simulink model "torqueBalancing2012b"  (Simulink 8.0)
settings: Solver=FixedStepDiscrete  StartTime=0.0  StopTime="CONFIG.SIMULATION_TIME "  FixedStep=CONFIG.Ts  RelTol=1e-3
InitFcn:
  | cd(fileparts(which(bdroot)));
  | initTorqueBalancing;
values from neighbouring files (symbols this model uses):
  WBT_modelName = 'matlabTorqueBalancing'    [initTorqueBalancing.m]
undefined symbols (not defined in the file or in its folder): bVectorConstraintsFeet, bVectorConstraintsLegs, CONFIG, ConstraintsMatrixFeet, ConstraintsMatrixLegs, DiscIntNeverNeededParam, gain, references, reg, ROBOT_DOF, ROBOT_DOF_FOR_SIMULINK, sat, SM, sm, WBT_robotName
libraries: WBToolboxLibrary x179, simulink x13
(part 1 of 4)
settings Model: Creator=daniele  LastModifiedBy=gnava
settings DebuggingCC: FcnCallInpInsideContextMsg=EnableAllAsWarning  FrameProcessingCompatibilityMsg=error
settings SFSimCC: SimParseCustomCode=off
settings CodeAppCC: CustomSymbolStrType=$N$R$M_T
settings GRTTargetCC: CodeReplacementLibrary=C89/C90 (ANSI)  CombineOutputUpdateFcns=off  GRTInterface=on

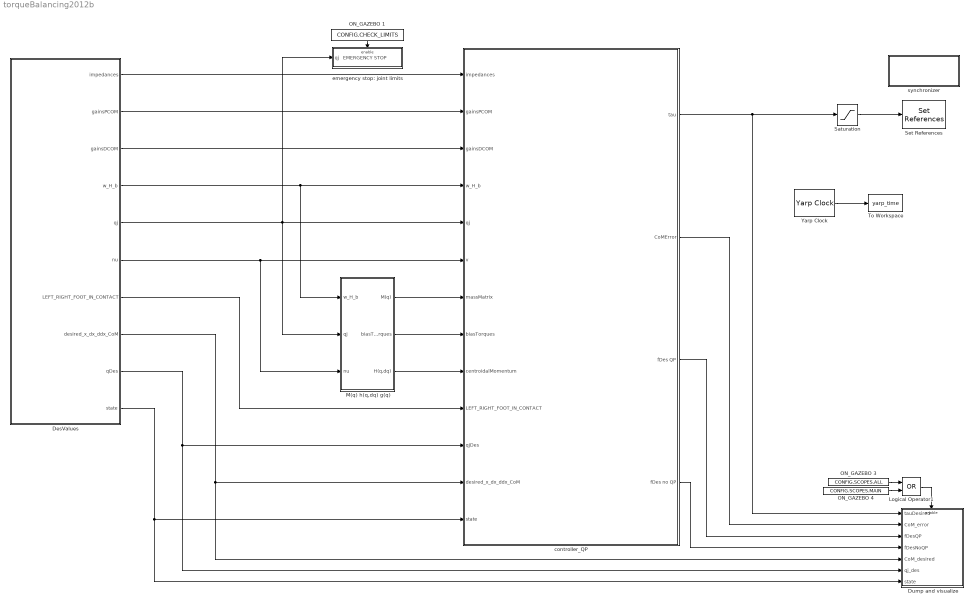
== system torqueBalancing2012b ==
  DesValues : Subsystem  Priority=-10
  Dump and visualize : Subsystem
  Logical Operator1 : Logic  Operator=OR  AllPortsSameDT=off  OutDataTypeStr=boolean
  M(q) h(q,dq) g(q) : Subsystem
  ON_GAZEBO 1 : Constant  Value=CONFIG.CHECK_LIMITS
  ON_GAZEBO 3 : Constant  Value=CONFIG.SCOPES.ALL
  ON_GAZEBO 4 : Constant  Value=CONFIG.SCOPES.MAIN
  Saturation : Saturate  UpperLimit=sat.torque  LowerLimit=-sat.torque
  Set References : WBToolboxLibrary/wholeBodyActuators/Set References  controlType=Torque  fullOrSubControl=Full  controlledJoints=''  robotName=WBT_robotName  localName=WBT_modelName  wbiFile=WBT_wbiFilename  wbiList=WBT_wbiList
  To Workspace : ToWorkspace  VariableName=yarp_time  SaveFormat=Structure With Time  SampleTime=-1
  Yarp Clock : WBToolboxLibrary/Utilities/Yarp Clock
  controller_QP : Subsystem
  emergency stop: joint limits : Subsystem
  synchronizer : Subsystem
      mask Display: disp('SYNCHRONIZER')
  wires:
  M(q) h(q,dq) g(q)/1(M(q)) -> controller_QP/7(massMatrix)
  DesValues/5(qj) -> emergency stop: joint limits/1(qj   EMERGENCY STOP), controller_QP/5(qj), M(q) h(q,dq) g(q)/2(qj)
  M(q) h(q,dq) g(q)/2(biasTorques) -> controller_QP/8(biasTorques)
  M(q) h(q,dq) g(q)/3(H(q,dq)) -> controller_QP/9(centroidalMomentum)
  controller_QP/1("tau ") -> Dump and visualize/1(tauDesired), Saturation/1
  controller_QP/2(CoMError) -> Dump and visualize/2(CoM_error)
  DesValues/9(qDes) -> Dump and visualize/6(qj_des), controller_QP/11(qjDes)
  DesValues/7(LEFT_RIGHT_FOOT_IN_CONTACT) -> controller_QP/10(LEFT_RIGHT_FOOT_IN_CONTACT)
  DesValues/8(desired_x_dx_ddx_CoM) -> controller_QP/12(desired_x_dx_ddx_CoM), Dump and visualize/5(CoM_desired)
  DesValues/1(impedances) -> controller_QP/1(impedances)
  Saturation/1 -> Set References/1
  DesValues/4(w_H_b) -> controller_QP/4(w_H_b), M(q) h(q,dq) g(q)/1(w_H_b)
  DesValues/6(nu) -> controller_QP/6(v), M(q) h(q,dq) g(q)/3(nu)
  Logical Operator1/1 -> Dump and visualize/Enable
  DesValues/10(state) -> Dump and visualize/7(state), controller_QP/13("state ")
  controller_QP/4(fDes no QP) -> Dump and visualize/4(fDesNoQP)
  controller_QP/3(fDes QP) -> Dump and visualize/3(fDesQP)
  ON_GAZEBO 1/1 -> emergency stop: joint limits/Enable
  ON_GAZEBO 3/1 -> Logical Operator1/1
  ON_GAZEBO 4/1 -> Logical Operator1/2
  DesValues/2(gainsPCOM) -> controller_QP/2(gainsPCOM)
  DesValues/3(gainsDCOM) -> controller_QP/3(gainsDCOM)
  Yarp Clock/1 -> To Workspace/1

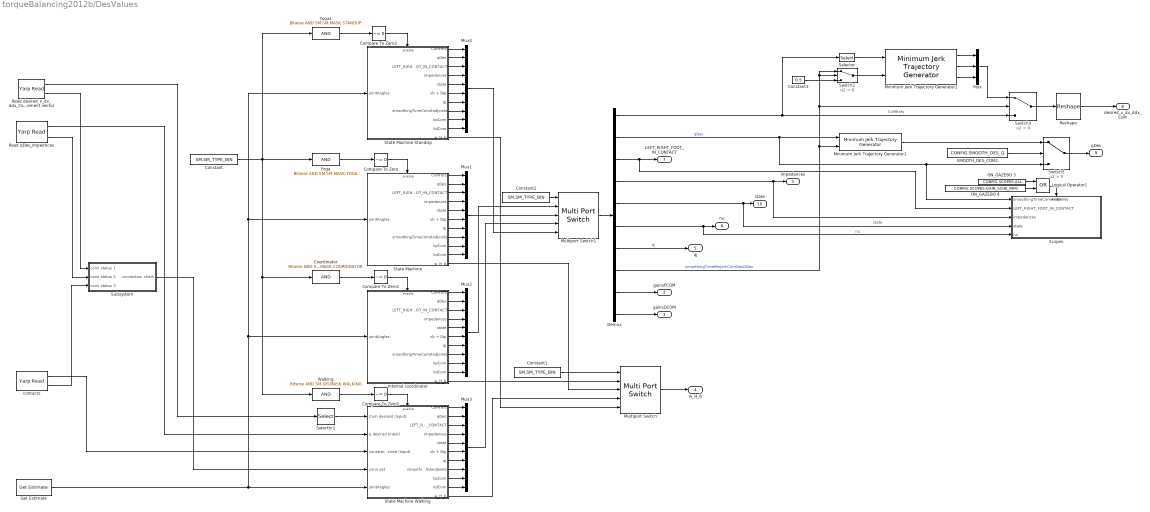
== system torqueBalancing2012b/DesValues ==
  Compare To Zero{,1..3} (4 alike) : simulink/Logic and Bit Operations/Compare To Zero  relop=~=  OutDataTypeStr=boolean
  Constant : Constant  Priority=-10  Value=SM.SM_TYPE_BIN  OutDataTypeStr=uint8
  Constant1 : Constant  Priority=-10  Value=SM.SM_TYPE_BIN  OutDataTypeStr=uint8
  Constant2 : Constant  Priority=-10  Value=SM.SM_TYPE_BIN  OutDataTypeStr=uint8
  Constant3 : Constant  Value=0.5
  Coordinator : simulink/Logic and Bit Operations/Bitwise Operator  logicop=AND  UseBitMask=on  BitMask=SM.SM.MASK.COORDINATOR  BitMaskRealWorld=Stored Integer
  Demux : Demux  Outputs=[9,ROBOT_DOF,2,ROBOT_DOF,1,ROBOT_DOF+6,ROBOT_DOF,1,3,3]
  Get Estimate : WBToolboxLibrary/wholeBodyStates/Get Estimate  estimateType=Joints Position  robotName=WBT_robotName  localName=WBT_modelName  wbiFile=WBT_wbiFilename  wbiList=WBT_wbiList
  Internal coordinator : Subsystem
  Logical Operator1 : Logic  Operator=OR  AllPortsSameDT=off  OutDataTypeStr=boolean
  Minimum Jerk Trajectory Generator1 : WBToolboxLibrary/Utilities/Minimum Jerk Trajectory Generator  externalSettlingTime=on  settlingTime=1  sampleTime=CONFIG.Ts  resetOnSettlingTime=off  firstDerivatives=off  secondDerivatives=off  explicitInitialValue=off
  Minimum Jerk Trajectory Generator2 : WBToolboxLibrary/Utilities/Minimum Jerk Trajectory Generator  externalSettlingTime=on  settlingTime=references.com.smoothingTime  sampleTime=CONFIG.Ts  resetOnSettlingTime=on  firstDerivatives=on  secondDerivatives=on  explicitInitialValue=off
  Multiport Switch : MultiPortSwitch  DataPortOrder=Specify indices  DataPortIndices={1, 2, 4, 6}
  Multiport Switch1 : MultiPortSwitch  DataPortOrder=Specify indices  DataPortIndices={1, 2, 4, 6}
  Mux : Mux  Inputs=3
  Mux{1..4} (4 alike) : Mux  Inputs=10
  ON_GAZEBO 3 : Constant  Value=CONFIG.SCOPES.ALL
  ON_GAZEBO 4 : Constant  Value=CONFIG.SCOPES.GAIN_SCHE_INFO
  Read desired_x_dx_ddx_CoM as 9 element vector : WBToolboxLibrary/Utilities/Yarp Read  portName=PORTS.COM_DES  signalSize=9  blocking=off  timestamp=off  autoconnect=off  errorOnConnection=on
  Read qDes_impednces : WBToolboxLibrary/Utilities/Yarp Read  portName=PORTS.Q_DES  signalSize=ROBOT_DOF  blocking=off  timestamp=off  autoconnect=off  errorOnConnection=on
  Reshape : Reshape  OutputDimensionality=Customize  OutputDimensions=[3,3]
  SMOOTH_DES_COM2 : Constant  Value=CONFIG.SMOOTH_DES_Q
  "Scopes  " : Subsystem
  Selector : Selector  InputPortWidth=9  IndexOptions=Index vector (dialog)  Indices=[1 2 3]  OutputSizes=1
  Selector1 : Selector  InputPortWidth=9  IndexOptions=Index vector (dialog)  Indices=[1 2 3]  OutputSizes=1
  State Machine : Subsystem  Priority=-100
  State Machine StandUp : Subsystem  Priority=-100
  State Machine Walking : Subsystem  Priority=-100
  Subsystem : Subsystem
  Switch1 : Switch  Criteria=u2 > Threshold
  Switch3 : Switch  Criteria=u2 > Threshold
  Switch5 : Switch  Criteria=u2 > Threshold
  Walking : simulink/Logic and Bit Operations/Bitwise Operator  logicop=AND  UseBitMask=on  BitMask=SM.SM.MASK.WALKING  BitMaskRealWorld=Stored Integer
  Yoga : simulink/Logic and Bit Operations/Bitwise Operator  logicop=AND  UseBitMask=on  BitMask=SM.SM.MASK.YOGA  BitMaskRealWorld=Stored Integer
  Yoga1 : simulink/Logic and Bit Operations/Bitwise Operator  logicop=AND  UseBitMask=on  BitMask=SM.SM.MASK.STANDUP  BitMaskRealWorld=Stored Integer
  contacts : WBToolboxLibrary/Utilities/Yarp Read  portName=['/' WBT_modelName '/constraints:i']  signalSize=2  blocking=off  timestamp=off  autoconnect=off  errorOnConnection=on
  impedances : Outport
  gainsPCOM : Outport  Port=2
  gainsDCOM : Outport  Port=3
  w_H_b : Outport  Port=4
  qj : Outport  Port=5
  nu : Outport  Port=6
  LEFT_RIGHT_FOOT_IN_CONTACT : Outport  Port=7
  desired_x_dx_ddx_CoM : Outport  Port=8
  qDes : Outport  Port=9
  state : Outport  Port=10
  wires:
  Read desired_x_dx_ddx_CoM as 9 element vector/2 -> Subsystem/1(conn status 1)
  Read desired_x_dx_ddx_CoM as 9 element vector/1 -> Selector1/1
  Reshape/1 -> desired_x_dx_ddx_CoM/1
  Read qDes_impednces/2 -> Subsystem/2(conn status 2)
  contacts/2 -> Subsystem/3(conn status 3)
  Switch3/1 -> Reshape/1
  SMOOTH_DES_COM2/1 -> Switch5/2
  Switch5/1 -> qDes/1
  Constant/1 -> Yoga1/1, Walking/1, Coordinator/1, Yoga/1
  State Machine/3(LEFT_RIGHT_FOOT_IN_CONTACT) -> Mux1/3
  State Machine/2(qDes) -> Mux1/2
  State Machine/1(CoMrefs) -> Mux1/1
  Internal coordinator/1(CoMrefs) -> Mux2/1
  Internal coordinator/2(qDes) -> Mux2/2
  Internal coordinator/3(LEFT_RIGHT_FOOT_IN_CONTACT) -> Mux2/3
  State Machine/4(impedances) -> Mux1/4
  Internal coordinator/4(impedances) -> Mux2/4
  State Machine/5(state) -> Mux1/5
  Internal coordinator/5(state) -> Mux2/5
  Internal coordinator/6(vb + Dqj) -> Mux2/6
  Internal coordinator/7(qj) -> Mux2/7
  State Machine/6(vb + Dqj) -> Mux1/6
  State Machine/7(qj) -> Mux1/7
  Demux/7 -> qj/1  "qj"
  State Machine Walking/4(impedances) -> Mux3/4
  State Machine Walking/3(LEFT_RIGHT_FOOT_IN_CONTACT) -> Mux3/3
  State Machine Walking/5(state) -> Mux3/5
  State Machine Walking/6(vb + Dqj) -> Mux3/6
  State Machine Walking/1(CoMrefs) -> Mux3/1
  State Machine Walking/7(qj) -> Mux3/7
  Coordinator/1 -> Compare To Zero1/1
  Yoga/1 -> Compare To Zero/1
  Walking/1 -> Compare To Zero2/1
  Mux3/1 -> Multiport Switch1/4
  Selector1/1 -> State Machine Walking/1(Com desired (input))
  Compare To Zero/1 -> State Machine/Enable
  Compare To Zero1/1 -> Internal coordinator/Enable
  Compare To Zero2/1 -> State Machine Walking/Enable
  Mux1/1 -> Multiport Switch1/3
  Mux2/1 -> Multiport Switch1/2
  State Machine/11(w_H_b) -> Multiport Switch/3
  Internal coordinator/11(w_H_b) -> Multiport Switch/2
  Read qDes_impednces/1 -> State Machine Walking/2(q desired (input))
  Subsystem/1(connection check) -> State Machine Walking/4(conn est)
  State Machine Walking/2(qDes) -> Mux3/2
  contacts/1 -> State Machine Walking/3(constraints desired (input))
  Multiport Switch/1 -> w_H_b/1
  Demux/5 -> state/1, "Scopes  "/4(state)  "state"
  Internal coordinator/8(smoothingTimeComAndJoints) -> Mux2/8
  State Machine Walking/8(smoothingTimeComAndJoints) -> Mux3/8
  State Machine/8(smoothingTimeComAndJoints) -> Mux1/8
  Demux/8 -> Switch1/1, Switch1/2, Switch3/2, Minimum Jerk Trajectory Generator1/2  "smoothingTimeMinJerkComDesQDes"
  Logical Operator1/1 -> "Scopes  "/Enable
  Demux/1 -> Selector/1, Switch3/3  "CoMRefs"
  Demux/2 -> Minimum Jerk Trajectory Generator1/1, "Scopes  "/1(smoothingTimeComAndJoints), Switch5/3  "qDes"
  Minimum Jerk Trajectory Generator1/1 -> Switch5/1
  ON_GAZEBO 3/1 -> Logical Operator1/1
  ON_GAZEBO 4/1 -> Logical Operator1/2
  Demux/6 -> nu/1, "Scopes  "/5(nu)  "nu"
  State Machine/9(kpCom) -> Mux1/9
  State Machine/10(kdCom) -> Mux1/10
  Internal coordinator/9(kpCom) -> Mux2/9
  Internal coordinator/10(kdCom) -> Mux2/10
  State Machine Walking/9(kpCom) -> Mux3/9
  State Machine Walking/10(kdCom) -> Mux3/10
  Multiport Switch1/1 -> Demux/1
  Demux/4 -> impedances/1, "Scopes  "/3(impedances)
  Demux/3 -> LEFT_RIGHT_FOOT_IN_CONTACT/1, "Scopes  "/2(LEFT_RIGHT_FOOT_IN_CONTACT)
  Demux/9 -> gainsPCOM/1
  Demux/10 -> gainsDCOM/1
  Constant1/1 -> Multiport Switch/1
  Constant2/1 -> Multiport Switch1/1
  Get Estimate/1 -> Internal coordinator/1(jointAngles), State Machine/1(jointAngles), State Machine StandUp/1(jointAngles), State Machine Walking/5(jointAngles)
  State Machine StandUp/3(LEFT_RIGHT_FOOT_IN_CONTACT) -> Mux4/3
  State Machine StandUp/2(qDes) -> Mux4/2
  State Machine StandUp/1(CoMrefs) -> Mux4/1
  State Machine StandUp/4(impedances) -> Mux4/4
  State Machine StandUp/5(state) -> Mux4/5
  State Machine StandUp/6(vb + Dqj) -> Mux4/6
  State Machine StandUp/7(qj) -> Mux4/7
  Yoga1/1 -> Compare To Zero3/1
  Compare To Zero3/1 -> State Machine StandUp/Enable
  State Machine StandUp/8(smoothingTimeComAndJoints) -> Mux4/8
  State Machine StandUp/9(kpCom) -> Mux4/9
  State Machine StandUp/10(kdCom) -> Mux4/10
  State Machine Walking/11(w_H_b) -> Multiport Switch/4
  State Machine StandUp/11(w_H_b) -> Multiport Switch/5
  Mux4/1 -> Multiport Switch1/5
  Minimum Jerk Trajectory Generator2/1 -> Mux/1
  Minimum Jerk Trajectory Generator2/2 -> Mux/2
  Minimum Jerk Trajectory Generator2/3 -> Mux/3
  Mux/1 -> Switch3/1
  Selector/1 -> Minimum Jerk Trajectory Generator2/1
  Switch1/1 -> Minimum Jerk Trajectory Generator2/2
  Constant3/1 -> Switch1/3

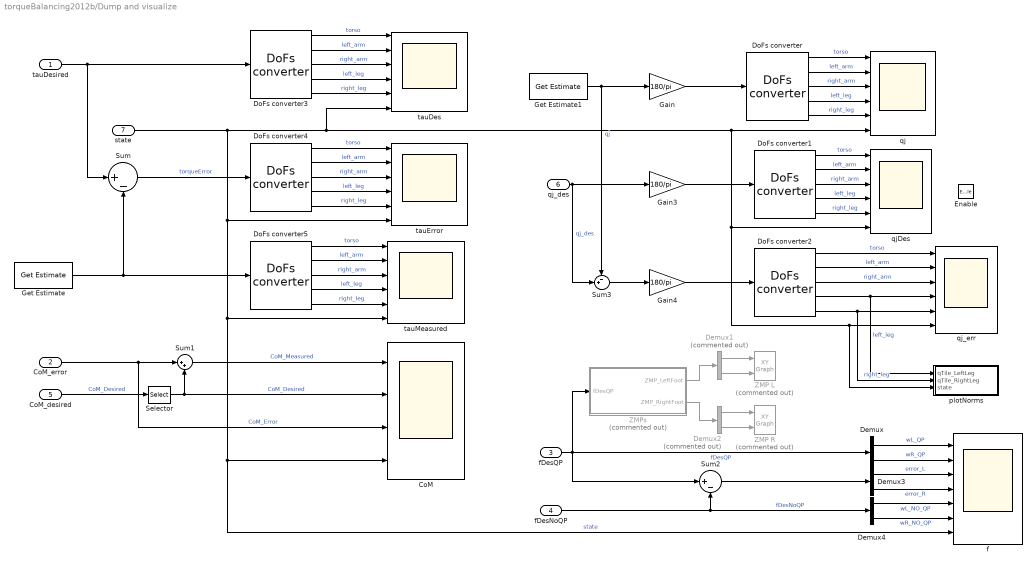
== system torqueBalancing2012b/Dump and visualize ==
  tauDesired : Inport
  CoM_error : Inport  Port=2
  fDesQP : Inport  Port=3
  fDesNoQP : Inport  Port=4
  CoM_desired : Inport  Port=5
  qj_des : Inport  Port=6
  state : Inport  Port=7
  Enable : EnablePort
  CoM : Scope  NumInputPorts=4
      settings: TimeRange=400  ShowLegends=on  MaxDataPoints=5000  SaveName=CoM_data  YMin=-0.20151~-0.19737~-0.11504~0.625  YMax=0.64612~0.73308~0.05288~4.375  SampleTime=-1
  Demux : Demux  Outputs=2
  Demux1 : Demux  Commented=on  Outputs=2
  Demux2 : Demux  Commented=on  Outputs=2
  Demux3 : Demux  Outputs=2
  Demux4 : Demux  Outputs=2
  DoFs converter{,1..5} (6 alike) : WBToolboxLibrary/Utilities/DoFs converter  yarp2WBIOption=From WBI to YARP  robotName=WBT_robotName  localName=WBT_modelName  wbiFile=WBT_wbiFilename  wbiList=WBT_wbiList
  Gain : Gain  Gain=180/pi
  Gain3 : Gain  Gain=180/pi
  Gain4 : Gain  Gain=180/pi
  Get Estimate : WBToolboxLibrary/wholeBodyStates/Get Estimate  estimateType=Joints Torque  robotName=WBT_robotName  localName=WBT_modelName  wbiFile=WBT_wbiFilename  wbiList=WBT_wbiList
  Get Estimate1 : WBToolboxLibrary/wholeBodyStates/Get Estimate  estimateType=Joints Position  robotName=WBT_robotName  localName=WBT_modelName  wbiFile=WBT_wbiFilename  wbiList=WBT_wbiList
  Selector : Selector  NumberOfDimensions=2  IndexOptions=Index vector (dialog),Index vector (dialog)  Indices=[1:3],1  OutputSizes=1,1
  Sum : Sum  Inputs=|+-
  Sum1 : Sum  Inputs=|++
  Sum2 : Sum  Inputs=|+-
  Sum3 : Sum  Inputs=-+|
  ZMP L : simulink/Sinks/XY Graph  Commented=on  xmin=gain.footSize(1,1)  xmax=gain.footSize(1,2)  ymin=gain.footSize(2,1)  ymax=gain.footSize(2,2)  st=-1
  ZMP R : simulink/Sinks/XY Graph  Commented=on  xmin=gain.footSize(1,1)  xmax=gain.footSize(1,2)  ymin=gain.footSize(2,1)  ymax=gain.footSize(2,2)  st=-1
  ZMPs : Subsystem  Commented=on
  f : Scope  NumInputPorts=7
      settings: TimeRange=40  MaxDataPoints=5000  SaveName=contactForces  YMin=-55.13342~-46.53033~-55.13342~-46.53033~-1.00000~-1.00000~0.375  YMax=287.07362~288.98447~287.07362~288.98447~1.00000~1.00000~6.625  SampleTime=-1
  plotNorms : Subsystem
  qj : Scope  NumInputPorts=6
      settings: TimeRange=40  ShowLegends=on  MaxDataPoints=5000  SaveName=qj_and_v  YMin=-22.0606~-111.86375~-112.26063~-123.37333~-122.0433~0.5  YMax=31.66267~49.03828~54.80749~108.78895~108.51909~5.5  SampleTime=-1
  qjDes : Scope  NumInputPorts=6
      settings: TimeRange=40  ShowLegends=on  MaxDataPoints=5000  SaveName=qj_and_v3  YMin=-3.30003~-109.64198~-109.55571~-122.73784~-122.54995~0.5  YMax=29.48051~49.50109~49.49151~110.23181~110.06609~5.5  SampleTime=-1
  qj_err : Scope  NumInputPorts=6
      settings: TimeRange=40  ShowLegends=on  MaxDataPoints=5000  SaveName=qj_and_v4  YMin=-36.22203~-18.04738~-18.01812~-53.76767~-55.62921~0.25  YMax=19.53985~12.8473~13.84456~64.5552~65.12215~7.75  SampleTime=-1
  tauDes : Scope  NumInputPorts=6
      settings: TimeRange=14  ShowLegends=on  MaxDataPoints=5000  SaveName=tauDes  YMin=-18.21791~-4.10899~-4.11637~-8.62065~-8.61496~0.9  YMax=2.04212~1.6382~1.63128~1.00779~0.97041~1.1  SampleTime=-1
  tauError : Scope  NumInputPorts=6
      settings: TimeRange=90  ShowLegends=on  MaxDataPoints=5000  SaveName=tauError  YMin=-11.13517~-2.53668~-2.28667~-29.03223~-17.07351~0.625  YMax=9.49915~1.99139~3.42607~28.25089~19.31802~4.375  SampleTime=-1
  tauMeasured : Scope  NumInputPorts=6
      settings: TimeRange=14  ShowLegends=on  MaxDataPoints=5000  SaveName=tauMeasured  YMin=-17.73267~-4.18816~-4.13415~-9.72494~-7.95735~0.9  YMax=2.55034~1.67903~1.65497~7.99033~7.48048~1.1  SampleTime=-1
  wires:
  CoM_error/1 -> Sum1/1, CoM/3  "CoM_Error"
  CoM_desired/1 -> Selector/1  "CoM_Desired"
  Sum1/1 -> CoM/1  "CoM_Measured"
  Get Estimate1/1 -> Sum3/1, Gain/1  "qj"
  Gain/1 -> DoFs converter/1
  DoFs converter/5 -> qj/5  "right_leg"
  DoFs converter/1 -> qj/1  "torso"
  DoFs converter/2 -> qj/2  "left_arm"
  DoFs converter/4 -> qj/4  "left_leg"
  DoFs converter/3 -> qj/3  "right_arm"
  fDesQP/1 -> Sum2/1, Demux/1, ZMPs/1(fDesQP)  "fDesQP"
  ZMPs/1(ZMP_LeftFoot) -> Demux1/1
  ZMPs/2(ZMP_RightFoot) -> Demux2/1
  Demux1/1 -> ZMP L/1
  Demux1/2 -> ZMP L/2
  Demux2/1 -> ZMP R/1
  Demux2/2 -> ZMP R/2
  Sum2/1 -> Demux3/1
  fDesNoQP/1 -> Demux4/1, Sum2/2  "fDesNoQP"
  tauDesired/1 -> DoFs converter3/1, Sum/1
  Get Estimate/1 -> Sum/2, DoFs converter5/1
  DoFs converter3/5 -> tauDes/5  "right_leg"
  DoFs converter3/1 -> tauDes/1  "torso"
  DoFs converter3/2 -> tauDes/2  "left_arm"
  DoFs converter3/4 -> tauDes/4  "left_leg"
  DoFs converter3/3 -> tauDes/3  "right_arm"
  DoFs converter4/5 -> tauError/5  "right_leg"
  DoFs converter4/1 -> tauError/1  "torso"
  DoFs converter4/2 -> tauError/2  "left_arm"
  DoFs converter4/4 -> tauError/4  "left_leg"
  DoFs converter4/3 -> tauError/3  "right_arm"
  Sum/1 -> DoFs converter4/1  "torqueError"
  DoFs converter5/5 -> tauMeasured/5  "right_leg"
  DoFs converter5/1 -> tauMeasured/1  "torso"
  DoFs converter5/2 -> tauMeasured/2  "left_arm"
  DoFs converter5/4 -> tauMeasured/4  "left_leg"
  DoFs converter5/3 -> tauMeasured/3  "right_arm"
  qj_des/1 -> Sum3/2, Gain3/1  "qj_des"
  Gain3/1 -> DoFs converter1/1
  DoFs converter1/5 -> qjDes/5  "right_leg"
  DoFs converter1/1 -> qjDes/1  "torso"
  DoFs converter1/2 -> qjDes/2  "left_arm"
  DoFs converter1/4 -> qjDes/4  "left_leg"
  DoFs converter1/3 -> qjDes/3  "right_arm"
  Gain4/1 -> DoFs converter2/1
  DoFs converter2/5 -> qj_err/5, plotNorms/2(qTile_RightLeg)  "right_leg"
  DoFs converter2/1 -> qj_err/1  "torso"
  DoFs converter2/2 -> qj_err/2  "left_arm"
  DoFs converter2/4 -> qj_err/4, plotNorms/1(qTile_LeftLeg)  "left_leg"
  DoFs converter2/3 -> qj_err/3  "right_arm"
  Sum3/1 -> Gain4/1
  Selector/1 -> Sum1/2, CoM/2  "CoM_Desired"
  state/1 -> tauDes/6, qj_err/6, plotNorms/3(state), qjDes/6, qj/6, f/7, CoM/4, tauMeasured/6, tauError/6  "state"
  Demux/1 -> f/1  "wL_QP"
  Demux/2 -> f/2  "wR_QP"
  Demux3/1 -> f/3  "error_L"
  Demux3/2 -> f/4  "error_R"
  Demux4/1 -> f/5  "wL_NO_QP"
  Demux4/2 -> f/6  "wR_NO_QP"

== system torqueBalancing2012b/M(q) h(q,dq) g(q) ==
  w_H_b : Inport
  qj : Inport  Port=2
  nu : Inport  Port=3
  Centroidal Momentum : WBToolboxLibrary/wholeBodyModel/Dynamics/Centroidal Momentum  robotName=WBT_robotName  localName=WBT_modelName  wbiFile=WBT_wbiFilename  wbiList=WBT_wbiList
  "CoM6D ->  CoMXYZ1" : Selector  InputPortWidth=6+ROBOT_DOF  IndexOptions=Index vector (dialog)  Indices=[7:6+ROBOT_DOF]  OutputSizes=1
  "CoM6D ->  CoMXYZ2" : Selector  InputPortWidth=6+ROBOT_DOF  IndexOptions=Index vector (dialog)  Indices=[1 2 3 4 5 6]  OutputSizes=1
  Get Bias Forces : WBToolboxLibrary/wholeBodyModel/Dynamics/Get Bias Forces  robotName=WBT_robotName  localName=WBT_modelName  wbiFile=WBT_wbiFilename  wbiList=WBT_wbiList  explicitGravity=off
  Mass Matrix : WBToolboxLibrary/wholeBodyModel/Dynamics/Mass Matrix  robotName=WBT_robotName  localName=WBT_modelName  wbiFile=WBT_wbiFilename  wbiList=WBT_wbiList
  M(q) : Outport
  biasTorques : Outport  Port=2
  H(q,dq) : Outport  Port=3
  wires:
  Mass Matrix/1 -> M(q)/1
  Centroidal Momentum/1 -> H(q,dq)/1
  Get Bias Forces/1 -> biasTorques/1
  w_H_b/1 -> Centroidal Momentum/1, Get Bias Forces/1, Mass Matrix/1
  qj/1 -> Centroidal Momentum/2, Get Bias Forces/2, Mass Matrix/2
  "CoM6D ->  CoMXYZ2"/1 -> Centroidal Momentum/3, Get Bias Forces/3
  "CoM6D ->  CoMXYZ1"/1 -> Get Bias Forces/4, Centroidal Momentum/4
  nu/1 -> "CoM6D ->  CoMXYZ1"/1, "CoM6D ->  CoMXYZ2"/1

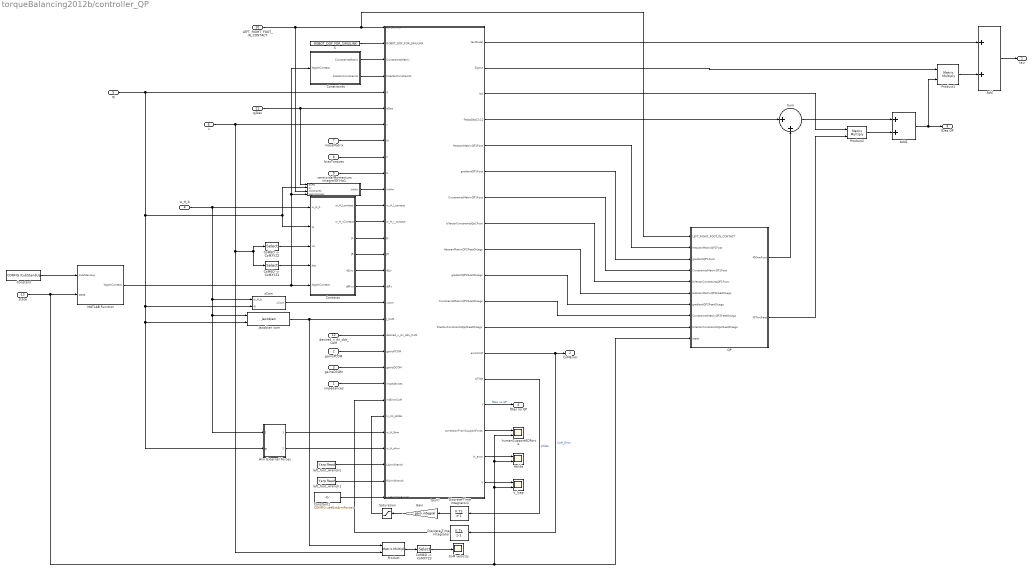
== system torqueBalancing2012b/controller_QP ==
  impedances : Inport
  gainsPCOM : Inport  Port=2
  gainsDCOM : Inport  Port=3
  w_H_b : Inport  Port=4
  qj : Inport  Port=5
  v : Inport  Port=6
  massMatrix : Inport  Port=7
  biasTorques : Inport  Port=8
  centroidalMomentum : Inport  Port=9
  LEFT_RIGHT_FOOT_IN_CONTACT : Inport  Port=10
  qjDes : Inport  Port=11
  desired_x_dx_ddx_CoM : Inport  Port=12
  "state " : Inport  Port=13
  "    5" : Constant  Value=ROBOT_DOF_FOR_SIMULINK
  Add : Sum
  Add1 : Sum
  Arm External Forces : Subsystem
  CoM velocity : Scope
      settings: TimeRange=auto  MaxDataPoints=5000  SaveName=CoMvelocity  YMin=-0.13469  YMax=0.38733  SampleTime=-1
  "CoM6D ->  CoMXYZ1" : Selector  InputPortWidth=6+ROBOT_DOF  IndexOptions=Index vector (dialog)  Indices=[7:6+ROBOT_DOF]  OutputSizes=1
  "CoM6D ->  CoMXYZ2" : Selector  InputPortWidth=6+ROBOT_DOF  IndexOptions=Index vector (dialog)  Indices=[1 2 3 4 5 6]  OutputSizes=1
  "CoM6D ->  CoMXYZ3" : Selector  InputPortWidth=6  IndexOptions=Index vector (dialog)  Indices=[1 2 3]  OutputSizes=1
  Constant : Constant  Value=CONFIG.iCubStandUp
  Constant1 : Constant  Value=CONFIG.useExtArmForces
  Constraints : Subsystem
  Contacts : Subsystem
  Discrete-Time Integrator : DiscreteIntegrator  InitialCondition=[0 0 0]  SampleTime=CONFIG.Ts  ICPrevOutput=DiscIntNeverNeededParam  ICPrevScaledInput=DiscIntNeverNeededParam
  Discrete-Time Integrator1 : DiscreteIntegrator  InitialCondition=zeros(ROBOT_DOF,1)  SampleTime=CONFIG.Ts  ICPrevOutput=DiscIntNeverNeededParam  ICPrevScaledInput=DiscIntNeverNeededParam
  Gain : Gain  Gain=gain.integral
  Htilde : Scope  NumInputPorts=2
      settings: TimeRange=auto  ShowLegends=on  MaxDataPoints=5000  SaveName=hTilde  YMin=-71.4251~0.75  YMax=58.40821~3.25  SampleTime=-1
  Jacobian com : WBToolboxLibrary/wholeBodyModel/Jacobians/Jacobian  frameName='com'  robotName=WBT_robotName  localName=WBT_modelName  wbiFile=WBT_wbiFilename  wbiList=WBT_wbiList
  MATLAB Function : MATLAB Function  TreatAsAtomicUnit=on
      settings: PermitHierarchicalResolution=ParametersOnly
  Product : Product  Multiplication=Matrix(*)
  Product1 : Product  Multiplication=Matrix(*)
  Product2 : Product  Multiplication=Matrix(*)
  QP : Subsystem
  Saturation : Saturate  UpperLimit=sat.integral  LowerLimit=-sat.integral
  Sum : Sum  Inputs=|++
  V_lyap : Scope  NumInputPorts=2
      settings: TimeRange=auto  ShowLegends=on  MaxDataPoints=5000  SaveName=V_lyap  YMin=-28009.24257~0.75  YMax=252083.18314~3.25  SampleTime=-1
  humanSupport6DForce : Scope  NumInputPorts=2
      settings: TimeRange=auto  ShowLegends=on  MaxDataPoints=5000  SaveName=helpingForcesOnH  YMin=-1.00000~0.75  YMax=1.00000~3.25  SampleTime=-1
  integralOf Hw1 : Subsystem
  left_foot_wrench1 : WBToolboxLibrary/Utilities/Yarp Read  portName=PORTS.RIGHT_ARM  signalSize=6  blocking=off  timestamp=off  autoconnect=on  errorOnConnection=on
  left_foot_wrench2 : WBToolboxLibrary/Utilities/Yarp Read  portName=PORTS.LEFT_ARM  signalSize=6  blocking=off  timestamp=off  autoconnect=on  errorOnConnection=on
  "tau(f) " : MATLAB Function  TreatAsAtomicUnit=on
      settings: PermitHierarchicalResolution=ParametersOnly
  xCom : Subsystem
  "tau " : Outport
  CoMError : Outport  Port=2
  fDes QP : Outport  Port=3
  fDes no QP : Outport  Port=4
  wires:
  LEFT_RIGHT_FOOT_IN_CONTACT/1 -> integralOf Hw1/3(constraints), QP/1(LEFT_RIGHT_FOOT_IN_CONTACT), "tau(f) "/1(constraints)
  Discrete-Time Integrator/1 -> "tau(f) "/24(intErrorCoM)
  "tau(f) "/13(errorCoM) -> Discrete-Time Integrator/1, CoMError/1  "CoM_Error"
  Discrete-Time Integrator1/1 -> Gain/1
  "tau(f) "/14(qTilde) -> Discrete-Time Integrator1/1  "qTilde"
  Gain/1 -> Saturation/1
  Saturation/1 -> "tau(f) "/25(ki_int_qtilde)
  qj/1 -> Arm External Forces/2(qj), Jacobian com/2, xCom/2(qj), integralOf Hw1/2(qj), Contacts/2(qj), "tau(f) "/5(q)
  qjDes/1 -> integralOf Hw1/1(qjDes), "tau(f) "/6(qDes)
  massMatrix/1 -> "tau(f) "/8(M)
  biasTorques/1 -> "tau(f) "/9(h)
  desired_x_dx_ddx_CoM/1 -> "tau(f) "/20(desired_x_dx_ddx_CoM)
  impedances/1 -> "tau(f) "/23(impedances)
  centroidalMomentum/1 -> "tau(f) "/10(H)
  Jacobian com/1 -> Product/1, "tau(f) "/19(J_CoM)
  "tau(f) "/5(HessianMatrixQP1Foot) -> QP/2(HessianMatrixQP1Foot)
  "tau(f) "/6(gradientQP1Foot) -> QP/3(gradientQP1Foot)
  "tau(f) "/9(HessianMatrixQP2FeetOrLegs) -> QP/6(HessianMatrixQP2FeetOrLegs)
  "tau(f) "/10(gradientQP2FeetOrLegs) -> QP/7(gradientQP2FeetOrLegs)
  "tau(f) "/11(ConstraintsMatrixQP2FeetOrLegs) -> QP/8(ConstraintsMatrixQP2FeetOrLegs)
  "tau(f) "/12(bVectorConstraintsQp2FeetOrLegs) -> QP/9(bVectorConstraintsQp2FeetOrLegs)
  "tau(f) "/4(fHdotDesC1C2) -> Sum/1
  QP/1(f0OneFoot) -> Sum/2
  Product1/1 -> Add/2
  "tau(f) "/1(tauModel) -> Add/1
  Add/1 -> "tau "/1
  Add1/1 -> fDes QP/1, Product1/2
  "    5"/1 -> "tau(f) "/2(ROBOT_DOF_FOR_SIMULINK)
  "tau(f) "/7(ConstraintsMatrixQP1Foot) -> QP/4(ConstraintsMatrixQP1Foot)
  "tau(f) "/8(bVectorConstraintsQp1Foot) -> QP/5(bVectorConstraintsQP1Foot)
  Sum/1 -> Add1/1
  Product2/1 -> Add1/2
  "tau(f) "/3(NA) -> Product2/1
  "tau(f) "/2(Sigma) -> Product1/1
  "tau(f) "/15(f) -> fDes no QP/1  "fDes no QP"
  integralOf Hw1/1(intHw) -> "tau(f) "/11(intHw)
  "state "/1 -> humanSupport6DForce/2, Htilde/2, V_lyap/2, QP/10(state), MATLAB Function/2(state)
  v/1 -> Product/2, "CoM6D ->  CoMXYZ2"/1, "CoM6D ->  CoMXYZ1"/1, "tau(f) "/7(v)
  Product/1 -> "CoM6D ->  CoMXYZ3"/1
  "CoM6D ->  CoMXYZ3"/1 -> CoM velocity/1
  gainsPCOM/1 -> "tau(f) "/21(gainsPCOM)
  gainsDCOM/1 -> "tau(f) "/22(gainsDCOM)
  w_H_b/1 -> Arm External Forces/1(w_H_b), Jacobian com/1, xCom/1(w_H_b), Contacts/1(w_H_b)
  QP/2(f0TwoFeet) -> Product2/2
  Constraints/1(ConstraintsMatrix) -> "tau(f) "/3(ConstraintsMatrix)
  Constraints/2(bVectorConstraints) -> "tau(f) "/4(bVectorConstraints)
  "CoM6D ->  CoMXYZ2"/1 -> Contacts/3(vb)
  "CoM6D ->  CoMXYZ1"/1 -> Contacts/4(dqj)
  Contacts/1(w_H_Lcontact) -> "tau(f) "/12(w_H_l_contact)
  Contacts/2(w_H_rContact) -> "tau(f) "/13(w_H_r_contact)
  Contacts/3(JL) -> "tau(f) "/14(JL)
  Contacts/4(JR) -> "tau(f) "/15(JR)
  Contacts/5(dJLnu) -> "tau(f) "/16(dJLv)
  Contacts/6(dJRnu) -> "tau(f) "/17(dJRv)
  Constant/1 -> MATLAB Function/1(icubStandup)
  MATLAB Function/1(legsInContact) -> Constraints/1(legsInContact), integralOf Hw1/4(legsInContact), Contacts/5(legsInContact)
  xCom/1(xCom) -> "tau(f) "/18(xcom)
  Arm External Forces/1(w_H_LArm) -> "tau(f) "/26(w_H_lArm)
  Arm External Forces/2(w_H_RArm) -> "tau(f) "/27(w_H_rArm)
  Constant1/1 -> "tau(f) "/30(useExtArmForces)
  left_foot_wrench2/1 -> "tau(f) "/28(LArmWrench)
  left_foot_wrench1/1 -> "tau(f) "/29(RArmWrench)
  "tau(f) "/16(correctionFromSupportForce) -> humanSupport6DForce/1
  "tau(f) "/17(H_error) -> Htilde/1
  "tau(f) "/18(V) -> V_lyap/1

== system torqueBalancing2012b/emergency stop: joint limits ==
  qj   EMERGENCY STOP : Inport
  Enable : EnablePort
  Assertion : Assertion
  Get Limits : WBToolboxLibrary/wholeBodyStates/Get Limits  limitsType=Position  robotName=WBT_robotName  localName=WBT_modelName  wbiFile=WBT_wbiFilename  wbiList=WBT_wbiList
  MATLAB Function : MATLAB Function  TreatAsAtomicUnit=on
      settings: PermitHierarchicalResolution=ParametersOnly
  index1 : Constant  Value=0.01  VectorParams1D=off
  wires:
  Get Limits/1 -> MATLAB Function/1(umin)
  Get Limits/2 -> MATLAB Function/2(umax)
  index1/1 -> MATLAB Function/4(tol)
  qj   EMERGENCY STOP/1 -> MATLAB Function/3(u)
  MATLAB Function/1(inRange) -> Assertion/1

== system torqueBalancing2012b/synchronizer ==
  GAZEBO_SYNCHRONIZER : Subsystem
  Logical Operator : Logic  Operator=NOT  AllPortsSameDT=off  OutDataTypeStr=boolean
  "ON_GAZEBO " : Constant  Value=CONFIG.ON_GAZEBO
  REAL_TIME_SYNC : Subsystem
  wires:
  Logical Operator/1 -> REAL_TIME_SYNC/Enable
  "ON_GAZEBO "/1 -> GAZEBO_SYNCHRONIZER/Enable, Logical Operator/1

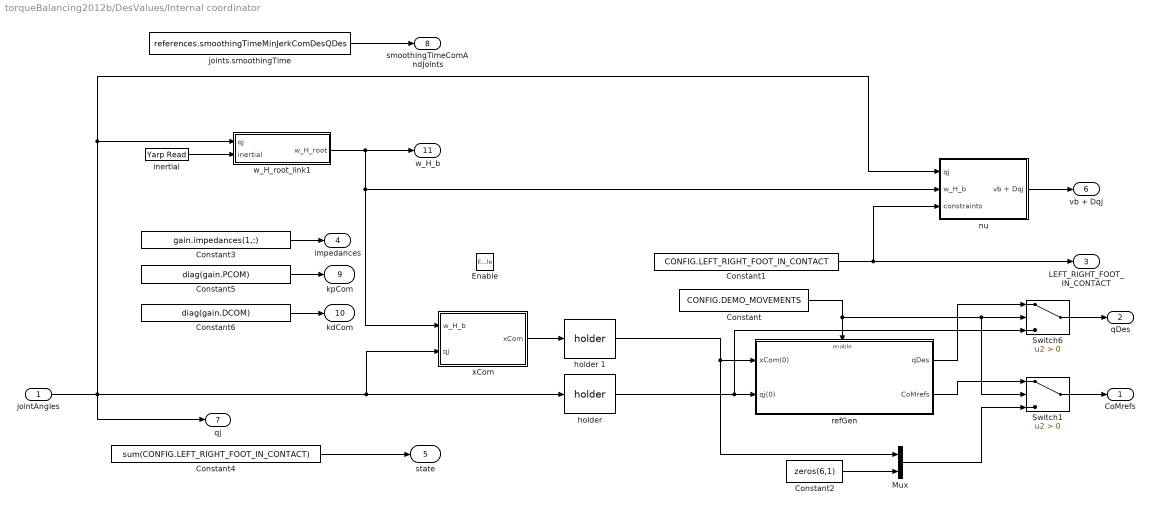
== system torqueBalancing2012b/DesValues/Internal coordinator ==
  jointAngles : Inport
  Enable : EnablePort
  Constant : Constant  Value=CONFIG.DEMO_MOVEMENTS
  Constant1 : Constant  Value=CONFIG.LEFT_RIGHT_FOOT_IN_CONTACT
  Constant2 : Constant  Value=zeros(6,1)
  Constant3 : Constant  Value=gain.impedances(1,:)
  Constant4 : Constant  Value=sum(CONFIG.LEFT_RIGHT_FOOT_IN_CONTACT)
  Constant5 : Constant  Value=diag(gain.PCOM)
  Constant6 : Constant  Value=diag(gain.DCOM)
  Mux : Mux  Inputs=2
  Switch1 : Switch  Criteria=u2 > Threshold
  Switch6 : Switch  Criteria=u2 > Threshold
  "holder " : WBToolboxLibrary/Utilities/holder 
  holder 1 : WBToolboxLibrary/Utilities/holder 
  inertial : WBToolboxLibrary/Utilities/Yarp Read  portName=PORTS.IMU  signalSize=12  blocking=off  timestamp=off  autoconnect=on  errorOnConnection=on
  joints.smoothingTime : Constant  Value=references.smoothingTimeMinJerkComDesQDes
  nu : Subsystem
  refGen : Subsystem
  w_H_root_link1 : Subsystem  mask{link_name='l_sole'}
      mask prompts: link_name "link name"
      mask help:
      | This block evaluates the homogeneous transformation between the world and the root link, i.e. ^wH_b. It assumes that the link specified by the variable 'link_name' has a constant position
      | w.r.t. an inertial frame, but it can rotate arbitrarily. This rotation is retrived from the IMU sensor.
      mask Display:
      | str = strrep(link_name, '_','\_');
      | port_label('output',1,['{}^{',str '}H_{root}'],'texmode','on')
      | clear str;
      | 
      | port_label('input',1,'q_j','texmode','on')
      | 
      | port_label('input',2,'inertial','texmode','on')
  xCom : Subsystem
  CoMrefs : Outport
  qDes : Outport  Port=2
  LEFT_RIGHT_FOOT_IN_CONTACT : Outport  Port=3
  impedances : Outport  Port=4
  state : Outport  Port=5
  vb + Dqj : Outport  Port=6
  qj : Outport  Port=7
  smoothingTimeComAndJoints : Outport  Port=8
  kpCom : Outport  Port=9
  kdCom : Outport  Port=10
  w_H_b : Outport  Port=11
  wires:
  Constant1/1 -> nu/3("constraints "), LEFT_RIGHT_FOOT_IN_CONTACT/1
  "holder "/1 -> refGen/2(qj(0)), Switch6/3
  Constant/1 -> Switch1/2, Switch6/2, refGen/Enable
  Switch6/1 -> qDes/1
  Switch1/1 -> CoMrefs/1
  refGen/1(qDes) -> Switch6/1
  refGen/2(CoMrefs) -> Switch1/1
  Mux/1 -> Switch1/3
  Constant2/1 -> Mux/2
  Constant3/1 -> impedances/1
  Constant4/1 -> state/1
  nu/1(vb + Dqj) -> vb + Dqj/1
  holder 1/1 -> Mux/1, refGen/1(xCom(0))
  w_H_root_link1/1(w_H_root) -> nu/2(w_H_b), xCom/1(w_H_b), w_H_b/1
  xCom/1(xCom) -> holder 1/1
  joints.smoothingTime/1 -> smoothingTimeComAndJoints/1
  jointAngles/1 -> "holder "/1, xCom/2(qj), qj/1, w_H_root_link1/1(qj), nu/1(qj)
  inertial/1 -> w_H_root_link1/2(inertial)
  Constant5/1 -> kpCom/1
  Constant6/1 -> kdCom/1

== system torqueBalancing2012b/DesValues/Scopes   ==
  smoothingTimeComAndJoints : Inport
  LEFT_RIGHT_FOOT_IN_CONTACT : Inport  Port=2
  impedances : Inport  Port=3
  state : Inport  Port=4
  nu : Inport  Port=5
  Enable : EnablePort
  Demux : Demux  Outputs=2
  DoFs converter : WBToolboxLibrary/Utilities/DoFs converter  yarp2WBIOption=From WBI to YARP  robotName=WBT_robotName  localName=WBT_modelName  wbiFile=WBT_wbiFilename  wbiList=WBT_wbiList
  DoFs converter1 : WBToolboxLibrary/Utilities/DoFs converter  yarp2WBIOption=From WBI to YARP  robotName=WBT_robotName  localName=WBT_modelName  wbiFile=WBT_wbiFilename  wbiList=WBT_wbiList
  Gain : Gain  Gain=180/pi
  Gain1 : Gain  Gain=180/pi
  Impedances(t) : Scope  NumInputPorts=6
      settings: TimeRange=auto  ShowLegends=on  MaxDataPoints=5000  SaveName=impedandesPlot  YMin=27.5~27.5~27.5~27.5~27.5~27.5  YMax=52.5~52.5~52.5~52.5~52.5~52.5  SampleTime=-1
  Left right foot in contact : Scope
      settings: TimeRange=auto  ShowLegends=on  MaxDataPoints=5000  SaveName=leftRightFootInContact  YMin=-0.09603  YMax=1.127  SampleTime=-1
  Selector1 : Selector  InputPortWidth=6+ROBOT_DOF  IndexOptions=Index vector (dialog)  Indices=[7:6+ROBOT_DOF]  OutputSizes=1
  Selector2 : Selector  InputPortWidth=6+ROBOT_DOF  IndexOptions=Index vector (dialog)  Indices=[1:6]  OutputSizes=1
  jointsSmoothingTime : Scope  NumInputPorts=2
      settings: TimeRange=auto  MaxDataPoints=5000  SaveName=smoothingTimes  YMin=-0.375~-0.375  YMax=13.375~13.375  SampleTime=-1
  linear and angular  base velocity : Scope  NumInputPorts=3
      settings: TimeRange=auto  ShowLegends=on  MaxDataPoints=5000  SaveName=baseVelocity  YMin=-0.04416~-19.05827~-0.5  YMax=0.05054~20.49714~14.5  SampleTime=-1
  "qjDot(t) " : Scope  NumInputPorts=6
      settings: TimeRange=60  ShowLegends=on  MaxDataPoints=5000  SaveName=dqj  YMin=-20.50153~-13.93091~-14.07118~-86.04652~-89.15901~-0.5  YMax=20.29706~17.04678~16.66387~63.96852~62.87068~14.5  SampleTime=-1
  wires:
  state/1 -> jointsSmoothingTime/2, "qjDot(t) "/6, linear and angular  base velocity/3, Impedances(t)/6  "state"
  LEFT_RIGHT_FOOT_IN_CONTACT/1 -> Left right foot in contact/1  "Left right foot in contact"
  impedances/1 -> DoFs converter/1
  smoothingTimeComAndJoints/1 -> jointsSmoothingTime/1  "smoothingTimeComAndJoints"
  DoFs converter/4 -> Impedances(t)/4  "left_leg"
  DoFs converter/5 -> Impedances(t)/5  "right_leg"
  DoFs converter/3 -> Impedances(t)/3  "right_arm"
  DoFs converter/1 -> Impedances(t)/1  "torso"
  DoFs converter/2 -> Impedances(t)/2  "left_arm"
  Selector1/1 -> Gain/1
  DoFs converter1/4 -> "qjDot(t) "/4  "left_leg"
  DoFs converter1/5 -> "qjDot(t) "/5  "right_leg"
  DoFs converter1/3 -> "qjDot(t) "/3  "right_arm"
  DoFs converter1/1 -> "qjDot(t) "/1  "torso"
  DoFs converter1/2 -> "qjDot(t) "/2  "left_arm"
  nu/1 -> Selector2/1, Selector1/1
  Selector2/1 -> Demux/1
  Demux/1 -> linear and angular  base velocity/1  "vb"
  Demux/2 -> Gain1/1  "wb"
  Gain/1 -> DoFs converter1/1
  Gain1/1 -> linear and angular  base velocity/2

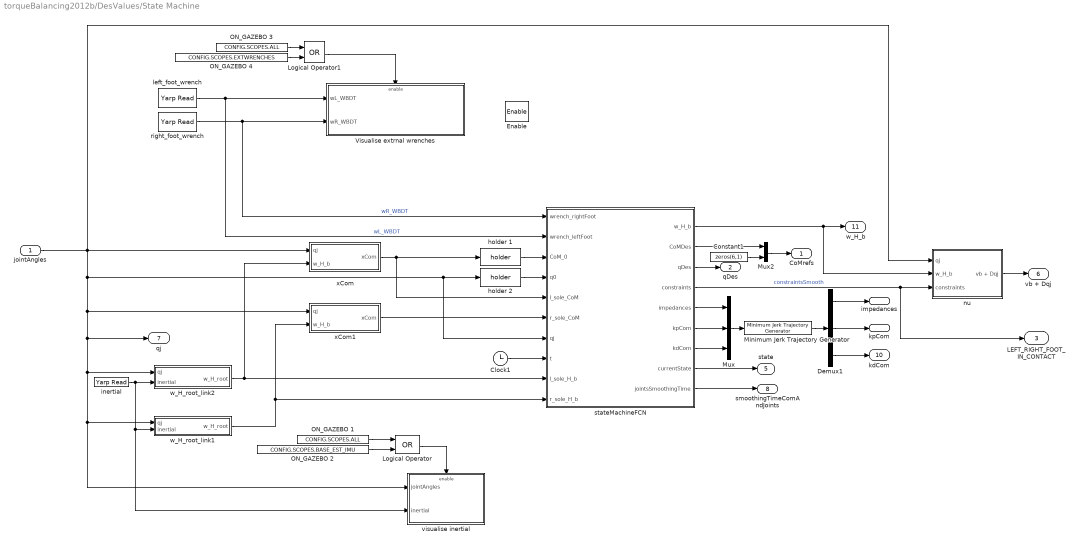
== system torqueBalancing2012b/DesValues/State Machine ==
  jointAngles : Inport
  Enable : EnablePort
  Clock1 : Clock
  Constant1 : Constant  Value=zeros(6,1)
  Demux1 : Demux  Outputs=[ROBOT_DOF,3,3]
  Logical Operator : Logic  Operator=OR  AllPortsSameDT=off  OutDataTypeStr=boolean
  Logical Operator1 : Logic  Operator=OR  AllPortsSameDT=off  OutDataTypeStr=boolean
  Minimum Jerk Trajectory Generator : WBToolboxLibrary/Utilities/Minimum Jerk Trajectory Generator  externalSettlingTime=off  settlingTime=gain.SmoothingTimeGainScheduling  sampleTime=CONFIG.Ts  resetOnSettlingTime=off  firstDerivatives=off  secondDerivatives=off  explicitInitialValue=off
  Mux : Mux  Inputs=3
  Mux2 : Mux  Inputs=2
  ON_GAZEBO 1 : Constant  Value=CONFIG.SCOPES.ALL
  ON_GAZEBO 2 : Constant  Value=CONFIG.SCOPES.BASE_EST_IMU
  ON_GAZEBO 3 : Constant  Value=CONFIG.SCOPES.ALL
  ON_GAZEBO 4 : Constant  Value=CONFIG.SCOPES.EXTWRENCHES
  "Visualise extrnal wrenches  " : Subsystem
  holder 1 : WBToolboxLibrary/Utilities/holder 
  holder 2 : WBToolboxLibrary/Utilities/holder 
  inertial : WBToolboxLibrary/Utilities/Yarp Read  portName=PORTS.IMU  signalSize=12  blocking=off  timestamp=off  autoconnect=on  errorOnConnection=on
  left_foot_wrench : WBToolboxLibrary/Utilities/Yarp Read  portName=PORTS.WBD_LEFTLEG_EE  signalSize=6  blocking=off  timestamp=off  autoconnect=on  errorOnConnection=on
  nu : Subsystem
  right_foot_wrench : WBToolboxLibrary/Utilities/Yarp Read  portName=PORTS.WBD_RIGHTLEG_EE  signalSize=6  blocking=off  timestamp=off  autoconnect=on  errorOnConnection=on
  stateMachineFCN : MATLAB Function  TreatAsAtomicUnit=on
      settings: PermitHierarchicalResolution=ParametersOnly
  visualise inertial : Subsystem
  w_H_root_link1 : Subsystem  mask{link_name='r_sole'}
      mask prompts: link_name "link name"
      mask help:
      | This block evaluates the homogeneous transformation between the world and the root link, i.e. ^wH_b. It assumes that the link specified by the variable 'link_name' has a constant position
      | w.r.t. an inertial frame, but it can rotate arbitrarily. This rotation is retrived from the IMU sensor.
      mask Display:
      | str = strrep(link_name, '_','\_');
      | port_label('output',1,['{}^{',str '}H_{root}'],'texmode','on')
      | clear str;
      | 
      | port_label('input',1,'q_j','texmode','on')
      | 
      | port_label('input',2,'inertial','texmode','on')
  w_H_root_link2 : Subsystem  mask{link_name='l_sole'}
      mask prompts: link_name "link name"
      mask help:
      | This block evaluates the homogeneous transformation between the world and the root link, i.e. ^wH_b. It assumes that the link specified by the variable 'link_name' has a constant position
      | w.r.t. an inertial frame, but it can rotate arbitrarily. This rotation is retrived from the IMU sensor.
      mask Display:
      | str = strrep(link_name, '_','\_');
      | port_label('output',1,['{}^{',str '}H_{root}'],'texmode','on')
      | clear str;
      | 
      | port_label('input',1,'q_j','texmode','on')
      | 
      | port_label('input',2,'inertial','texmode','on')
  xCom : Subsystem
  xCom1 : Subsystem
  CoMrefs : Outport
  qDes : Outport  Port=2
  LEFT_RIGHT_FOOT_IN_CONTACT : Outport  Port=3
  impedances : Outport  Port=4
  state : Outport  Port=5
  vb + Dqj : Outport  Port=6
  qj : Outport  Port=7
  smoothingTimeComAndJoints : Outport  Port=8
  kpCom : Outport  Port=9
  kdCom : Outport  Port=10
  w_H_b : Outport  Port=11
  wires:
  right_foot_wrench/1 -> "Visualise extrnal wrenches  "/2(wR_WBDT), stateMachineFCN/1(wrench_rightFoot)  "wR_WBDT"
  xCom/1(xCom) -> stateMachineFCN/5(l_sole_CoM), holder 1/1
  holder 1/1 -> stateMachineFCN/3(CoM_0)
  holder 2/1 -> stateMachineFCN/4(q0)
  Clock1/1 -> stateMachineFCN/8(t)
  stateMachineFCN/3(qDes) -> qDes/1
  stateMachineFCN/2(CoMDes) -> Mux2/1
  Mux2/1 -> CoMrefs/1
  Constant1/1 -> Mux2/2
  stateMachineFCN/8(currentState) -> state/1
  stateMachineFCN/4(constraints) -> LEFT_RIGHT_FOOT_IN_CONTACT/1, nu/3("constraints ")  "constraintsSmooth"
  left_foot_wrench/1 -> "Visualise extrnal wrenches  "/1(wL_WBDT), stateMachineFCN/2(wrench_leftFoot)  "wL_WBDT"
  stateMachineFCN/1(w_H_b) -> w_H_b/1, nu/2(w_H_b)
  xCom1/1(xCom) -> stateMachineFCN/6(r_sole_CoM)
  nu/1(vb + Dqj) -> vb + Dqj/1
  w_H_root_link2/1(w_H_root) -> stateMachineFCN/9(l_sole_H_b), xCom/2(w_H_b)
  w_H_root_link1/1(w_H_root) -> stateMachineFCN/10(r_sole_H_b), xCom1/2(w_H_b)
  jointAngles/1 -> w_H_root_link2/1(qj), w_H_root_link1/1(qj), visualise inertial/1(jointAngles), qj/1, xCom1/1(qj), stateMachineFCN/7(qj), holder 2/1, nu/1(qj), xCom/1(qj)
  inertial/1 -> w_H_root_link2/2(inertial), w_H_root_link1/2(inertial), visualise inertial/2(inertial)
  stateMachineFCN/9(jointsSmoothingTime) -> smoothingTimeComAndJoints/1
  Logical Operator1/1 -> "Visualise extrnal wrenches  "/Enable
  ON_GAZEBO 1/1 -> Logical Operator/1
  ON_GAZEBO 2/1 -> Logical Operator/2
  Logical Operator/1 -> visualise inertial/Enable
  ON_GAZEBO 3/1 -> Logical Operator1/1
  ON_GAZEBO 4/1 -> Logical Operator1/2
  stateMachineFCN/6(kpCom) -> Mux/2
  Demux1/3 -> kdCom/1
  stateMachineFCN/7(kdCom) -> Mux/3
  stateMachineFCN/5(impedances) -> Mux/1
  Mux/1 -> Minimum Jerk Trajectory Generator/1
  Minimum Jerk Trajectory Generator/1 -> Demux1/1
  Demux1/1 -> impedances/1
  Demux1/2 -> kpCom/1

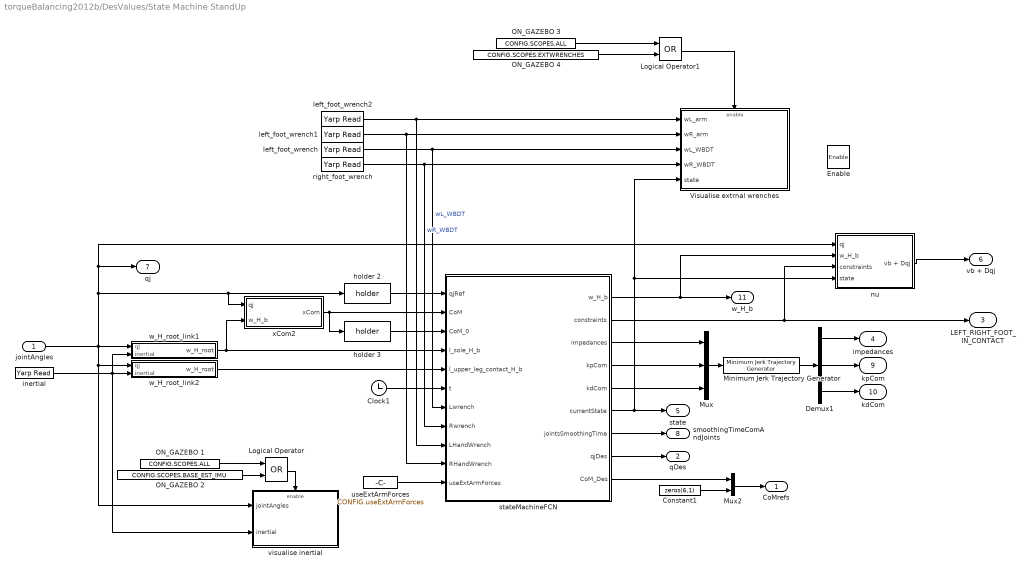
== system torqueBalancing2012b/DesValues/State Machine StandUp ==
  jointAngles : Inport
  Enable : EnablePort
  Clock1 : Clock
  Constant1 : Constant  Value=zeros(6,1)
  Demux1 : Demux  Outputs=[ROBOT_DOF,3,3]
  Logical Operator : Logic  Operator=OR  AllPortsSameDT=off  OutDataTypeStr=boolean
  Logical Operator1 : Logic  Operator=OR  AllPortsSameDT=off  OutDataTypeStr=boolean
  Minimum Jerk Trajectory Generator : WBToolboxLibrary/Utilities/Minimum Jerk Trajectory Generator  externalSettlingTime=off  settlingTime=gain.SmoothingTimeGainScheduling  sampleTime=CONFIG.Ts  resetOnSettlingTime=off  firstDerivatives=off  secondDerivatives=off  explicitInitialValue=off
  Mux : Mux  Inputs=3
  Mux2 : Mux  Inputs=2
  ON_GAZEBO 1 : Constant  Value=CONFIG.SCOPES.ALL
  ON_GAZEBO 2 : Constant  Value=CONFIG.SCOPES.BASE_EST_IMU
  ON_GAZEBO 3 : Constant  Value=CONFIG.SCOPES.ALL
  ON_GAZEBO 4 : Constant  Value=CONFIG.SCOPES.EXTWRENCHES
  "Visualise extrnal wrenches  " : Subsystem
  holder 2 : WBToolboxLibrary/Utilities/holder 
  holder 3 : WBToolboxLibrary/Utilities/holder 
  inertial : WBToolboxLibrary/Utilities/Yarp Read  portName=PORTS.IMU  signalSize=12  blocking=off  timestamp=off  autoconnect=on  errorOnConnection=on
  left_foot_wrench : WBToolboxLibrary/Utilities/Yarp Read  portName=PORTS.WBD_LEFTLEG_EE  signalSize=6  blocking=off  timestamp=off  autoconnect=on  errorOnConnection=on
  left_foot_wrench1 : WBToolboxLibrary/Utilities/Yarp Read  portName=PORTS.RIGHT_ARM  signalSize=6  blocking=off  timestamp=off  autoconnect=on  errorOnConnection=on
  left_foot_wrench2 : WBToolboxLibrary/Utilities/Yarp Read  portName=PORTS.LEFT_ARM  signalSize=6  blocking=off  timestamp=off  autoconnect=on  errorOnConnection=on
  nu : Subsystem
  right_foot_wrench : WBToolboxLibrary/Utilities/Yarp Read  portName=PORTS.WBD_RIGHTLEG_EE  signalSize=6  blocking=off  timestamp=off  autoconnect=on  errorOnConnection=on
  stateMachineFCN : MATLAB Function  TreatAsAtomicUnit=on
      settings: PermitHierarchicalResolution=ParametersOnly
  useExtArmForces : Constant  Value=CONFIG.useExtArmForces
  visualise inertial : Subsystem
  w_H_root_link1 : Subsystem  mask{link_name='l_sole'}
      mask prompts: link_name "link name"
      mask help:
      | This block evaluates the homogeneous transformation between the world and the root link, i.e. ^wH_b. It assumes that the link specified by the variable 'link_name' has a constant position
      | w.r.t. an inertial frame, but it can rotate arbitrarily. This rotation is retrived from the IMU sensor.
      mask Display:
      | str = strrep(link_name, '_','\_');
      | port_label('output',1,['{}^{',str '}H_{root}'],'texmode','on')
      | clear str;
      | 
      | port_label('input',1,'q_j','texmode','on')
      | 
      | port_label('input',2,'inertial','texmode','on')
  w_H_root_link2 : Subsystem  mask{link_name='l_upper_leg_contact'}
      mask prompts: link_name "link name"
      mask help:
      | This block evaluates the homogeneous transformation between the world and the root link, i.e. ^wH_b. It assumes that the link specified by the variable 'link_name' has a constant position
      | w.r.t. an inertial frame, but it can rotate arbitrarily. This rotation is retrived from the IMU sensor.
      mask Display:
      | str = strrep(link_name, '_','\_');
      | port_label('output',1,['{}^{',str '}H_{root}'],'texmode','on')
      | clear str;
      | 
      | port_label('input',1,'q_j','texmode','on')
      | 
      | port_label('input',2,'inertial','texmode','on')
  xCom2 : Subsystem
  CoMrefs : Outport
  qDes : Outport  Port=2
  LEFT_RIGHT_FOOT_IN_CONTACT : Outport  Port=3
  impedances : Outport  Port=4
  state : Outport  Port=5
  vb + Dqj : Outport  Port=6
  qj : Outport  Port=7
  smoothingTimeComAndJoints : Outport  Port=8
  kpCom : Outport  Port=9
  kdCom : Outport  Port=10
  w_H_b : Outport  Port=11
  wires:
  right_foot_wrench/1 -> "Visualise extrnal wrenches  "/4(wR_WBDT), stateMachineFCN/8(Rwrench)  "wR_WBDT"
  Mux2/1 -> CoMrefs/1
  Constant1/1 -> Mux2/2
  left_foot_wrench/1 -> stateMachineFCN/7(Lwrench), "Visualise extrnal wrenches  "/3(wL_WBDT)  "wL_WBDT"
  nu/1(vb + Dqj) -> vb + Dqj/1
  jointAngles/1 -> w_H_root_link2/1(qj), visualise inertial/1(jointAngles), qj/1, nu/1(qj), holder 2/1, xCom2/1(qj), w_H_root_link1/1(qj)
  inertial/1 -> w_H_root_link2/2(inertial), visualise inertial/2(inertial), w_H_root_link1/2(inertial)
  Logical Operator1/1 -> "Visualise extrnal wrenches  "/Enable
  ON_GAZEBO 1/1 -> Logical Operator/1
  ON_GAZEBO 2/1 -> Logical Operator/2
  Logical Operator/1 -> visualise inertial/Enable
  ON_GAZEBO 3/1 -> Logical Operator1/1
  ON_GAZEBO 4/1 -> Logical Operator1/2
  Demux1/3 -> kdCom/1
  Mux/1 -> Minimum Jerk Trajectory Generator/1
  Minimum Jerk Trajectory Generator/1 -> Demux1/1
  Demux1/1 -> impedances/1
  Demux1/2 -> kpCom/1
  w_H_root_link1/1(w_H_root) -> xCom2/2(w_H_b), stateMachineFCN/4(l_sole_H_b)
  w_H_root_link2/1(w_H_root) -> stateMachineFCN/5(l_upper_leg_contact_H_b)
  Clock1/1 -> stateMachineFCN/6(t)
  stateMachineFCN/3(impedances) -> Mux/1
  stateMachineFCN/4(kpCom) -> Mux/2
  stateMachineFCN/5(kdCom) -> Mux/3
  stateMachineFCN/7(jointsSmoothingTime) -> smoothingTimeComAndJoints/1
  stateMachineFCN/2(constraints) -> LEFT_RIGHT_FOOT_IN_CONTACT/1, nu/3("constraints ")
  holder 2/1 -> stateMachineFCN/1(qjRef)
  stateMachineFCN/8(qjDes) -> qDes/1
  xCom2/1(xCom) -> holder 3/1, stateMachineFCN/2(CoM)
  holder 3/1 -> stateMachineFCN/3(CoM_0)
  stateMachineFCN/9(CoM_Des) -> Mux2/1
  stateMachineFCN/1(w_H_b) -> w_H_b/1, nu/2(w_H_b)
  left_foot_wrench1/1 -> stateMachineFCN/10(RHandWrench), "Visualise extrnal wrenches  "/2(wR_arm)
  left_foot_wrench2/1 -> stateMachineFCN/9(LHandWrench), "Visualise extrnal wrenches  "/1(wL_arm)
  useExtArmForces/1 -> stateMachineFCN/11(useExtArmForces)
  stateMachineFCN/6(currentState) -> state/1, nu/4("state "), "Visualise extrnal wrenches  "/5(state)
